simulink model "Function_1"  (R2021a)
settings: Solver=VariableStepAuto  StartTime=0.0  StopTime=10.0  RelTol=1e-3
settings Model: Creator=nicol  LastModifiedBy=nicol

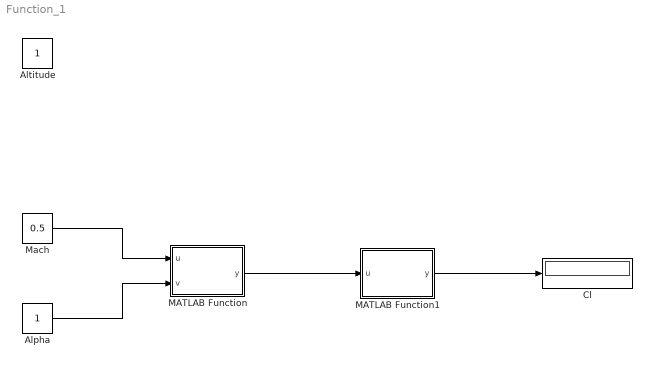
== system Function_1 ==
  Alpha : Constant
  Altitude : Constant
  Cl : Display
  MATLAB Function : MATLAB Function  TreatAsAtomicUnit=on
  MATLAB Function1 : MATLAB Function  TreatAsAtomicUnit=on
  Mach : Constant  Value=0.5  OutMin=0  OutMax=0.9
  wires:
  MATLAB Function/1(y) -> MATLAB Function1/1(u)
  Mach/1 -> MATLAB Function/1(u)
  Alpha/1 -> MATLAB Function/2(v)
  MATLAB Function1/1(y) -> Cl/1

== matlab function Function_1/MATLAB Function ==
  data: u input; y output; v input
function y = fcn(u,v)
% First method, linearized theory for a thin plate
y = ((2*pi*(v*2*pi)/360)/(sqrt(1-u^2)))*13500/(2*pi*52^2);

== matlab function Function_1/MATLAB Function1 ==
  data: u input; y output
function y = fcn(u)
% Second method, lift partition
y = u*2;
